simulink model "test"  (R2023b)
settings: Solver=FixedStepAuto  StartTime=0.0  StopTime=10.0  FixedStep=5e-8  RelTol=1e-3
undefined symbols (not defined in the file): powergui, sps_lib
libraries: spsMosfetLib x6, mcbcontrolslib x4, dspfdesign x3, slpidlib x3, simulink x2, spsDCVoltageSourceLib x1, spsPermanentMagnetSynchronousMachineLib x1, spsSawtoothGeneratorLib x1
settings Model: Creator=LZQ  LastModifiedBy=LZQ

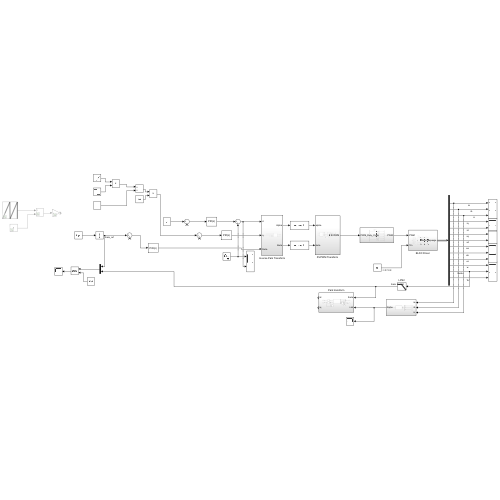
[thumbnail: Simulink's stored preview of the top-level diagram]
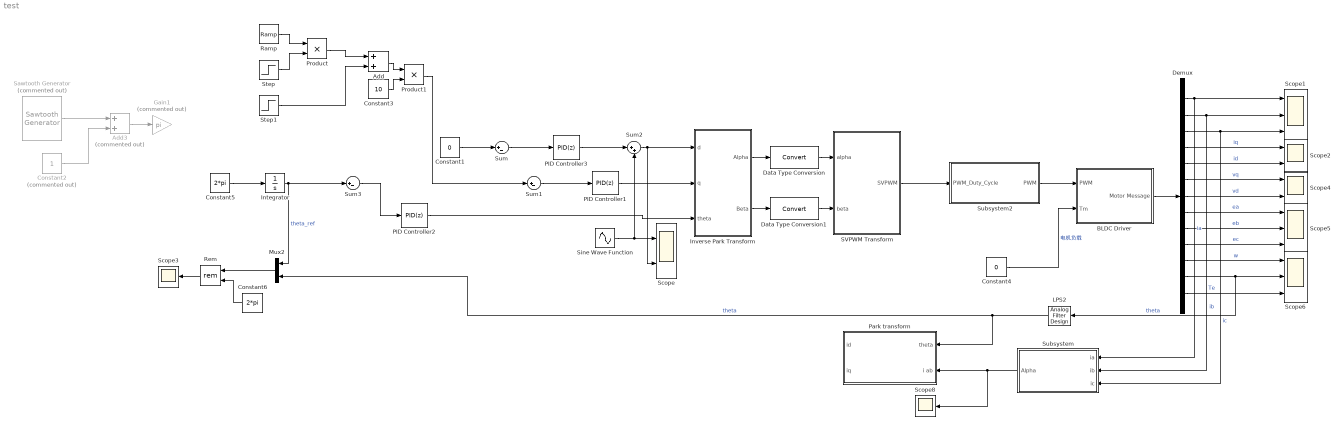
== system test ==
  Add : Sum
  Add3 : Sum  Commented=on
  BLDC Driver : Subsystem
  Constant1 : Constant  Value=0
  Constant2 : Constant  Commented=on
  Constant3 : Constant  Value=10
  Constant4 : Constant  Value=0
  Constant5 : Constant  Value=2*pi
  Constant6 : Constant  Value=2*pi
  Data Type Conversion : DataTypeConversion  SaturateOnIntegerOverflow=off  RndMeth=Floor
  Data Type Conversion1 : DataTypeConversion  SaturateOnIntegerOverflow=off  RndMeth=Floor
  Demux : Demux  Outputs=13
  Gain1 : Gain  Commented=on  Gain=pi
  Integrator : Integrator
  Inverse Park Transform : Subsystem
  LPS2 : dspfdesign/Analog Filter Design  method=Butterworth  filttype=Lowpass  N=8  Wlo=30  Whi=80  Rp=2  Rs=40
  Mux2 : Mux  Inputs=2
  PID Controller1 : slpidlib/PID Controller  Controller=PID  Form=Parallel  TimeDomain=Discrete-time  UseExternalTs=off  SampleTime=0.0005  IntegratorMethod=Forward Euler  FilterMethod=Forward Euler  ControllerParametersSource=internal  P=0.04  I=0.01  UseKiTs=off  D=0.008  N=100  UseFilter=on  TunerSelectOption=Transfer Function Based (PID Tuner App)  InitialConditionSource=internal  InitialConditionForIntegrator=0  InitialConditionForFilter=0  DifferentiatorICPrevScaledInput=0  ExternalReset=none  TrackingMode=off  Kt=1  LimitOutput=off  SatLimitsSource=internal  UpperSaturationLimit=inf  LowerSaturationLimit=-inf  LinearizeAsGain=on  AntiWindupMode=none  Kb=1  LimitIntegrator=off  UpperIntegratorSaturationLimit=inf  LowerIntegratorSaturationLimit=-inf  POutMin=[]  POutMax=[]  IOutMin=[-5]  IOutMax=[5]  DOutMin=[]  DOutMax=[]  NOutMin=[]  NOutMax=[]  SumOutMin=[-10]  SumOutMax=[10]  SaturationOutMin=[]  SaturationOutMax=[]  PParamMin=[]  PParamMax=[]  IParamMin=[]  IParamMax=[]  DParamMin=[]  DParamMax=[]  NParamMin=[]  NParamMax=[]  KbParamMin=[]  KbParamMax=[]  KtParamMin=[]  KtParamMax=[]  KbOutMin=[]  KbOutMax=[]  KtOutMin=[]  KtOutMax=[]  IntegratorOutMin=[]  IntegratorOutMax=[]  FilterOutMin=[]  FilterOutMax=[]  SumI1OutMin=[]  SumI1OutMax=[]  SumI2OutMin=[]  SumI2OutMax=[]  SumI3OutMin=[]  SumI3OutMax=[]  SumI4OutMin=[]  SumI4OutMax=[]  SumDOutMin=[]  SumDOutMax=[]  DifferentiatorOutMin=[]  DifferentiatorOutMax=[]  FilterDiffOutCoefMin=[]  FilterDiffOutCoefMax=[]  ReciprocalOutMin=[]  ReciprocalOutMax=[]  SumDenOutMin=[]  SumDenOutMax=[]  SumNumOutMin=[]  SumNumOutMax=[]  DivideOutMin=[]  DivideOutMax=[]  UdiffTsProdOutMin=[]  UdiffTsProdOutMax=[]  NTsProdOutMin=[]  NTsProdOutMax=[]  UintegralTsProdOutMin=[]  UintegralTsProdOutMax=[]  UngainTsProdOutMin=[]  UngainTsProdOutMax=[]  ClampingZeroOutDataTypeStr=Inherit: Inherit via back propagation  ClampingZeroOutMin=[]  ClampingZeroOutMax=[]  FilterDenConstantOutDataTypeStr=Inherit: Inherit via back propagation  FilterDenConstantOutMin=[]  FilterDenConstantOutMax=[]  PCopyOutDataTypeStr=Inherit: Inherit via back propagation  PCopyOutMin=[]  PCopyOutMax=[]  NCopyOutDataTypeStr=Inherit: Inherit via back propagation  NCopyOutMin=[]  NCopyOutMax=[]  IntegratorContinuousStateAttributes=''  IntegratorStateMustResolveToSignalObject=off  IntegratorRTWStateStorageClass=Auto  FilterContinuousStateAttributes=''  FilterStateMustResolveToSignalObject=off  FilterRTWStateStorageClass=Auto  ParallelPVariant=InternalParameters  IdealPVariant=Disabled  IVariant=InternalParameters  DVariant=InternalParameters  IntegratorVariant=Discrete  SatVariant=Disabled  AWVariant=Passthrough  PCopyVariant=Disabled  TRVariant=Disabled  FdbkBlocksVariant=Forward  IdealPFdbkVariant=Disabled  SatFdbkVariant=Disabled  DerivativeFilterVariant=ForwardEulerFilter  NVariant=InternalParameters  NCopyVariant=Disabled  FilterICVariant=InternalICsFilter  IntegratorICVariant=InternalICs  ExternalResetVariant=Disabled  TRSumVariant=Passthrough  SumFdbkVariant=Disabled  SumVariant=Sum_PID  TsampFilterVariant=InternalTs  TsampNgainVariant=Passthrough  TsampIntegralVariant=Disabled_SignalSpec  ExternalSaturationOutDataTypeStr=Inherit: Same as second input
  PID Controller2 : slpidlib/PID Controller  Controller=PID  Form=Parallel  TimeDomain=Discrete-time  UseExternalTs=off  SampleTime=0.0005  IntegratorMethod=Forward Euler  FilterMethod=Forward Euler  ControllerParametersSource=internal  P=0.1  I=0.04  UseKiTs=off  D=0  N=100  UseFilter=on  TunerSelectOption=Transfer Function Based (PID Tuner App)  InitialConditionSource=internal  InitialConditionForIntegrator=0  InitialConditionForFilter=0  DifferentiatorICPrevScaledInput=0  ExternalReset=none  TrackingMode=off  Kt=1  LimitOutput=off  SatLimitsSource=internal  UpperSaturationLimit=inf  LowerSaturationLimit=-inf  LinearizeAsGain=on  AntiWindupMode=none  Kb=1  LimitIntegrator=off  UpperIntegratorSaturationLimit=inf  LowerIntegratorSaturationLimit=-inf  POutMin=[]  POutMax=[]  IOutMin=[]  IOutMax=[]  DOutMin=[]  DOutMax=[]  NOutMin=[]  NOutMax=[]  SumOutMin=[]  SumOutMax=[]  SaturationOutMin=[]  SaturationOutMax=[]  PParamMin=[]  PParamMax=[]  IParamMin=[]  IParamMax=[]  DParamMin=[]  DParamMax=[]  NParamMin=[]  NParamMax=[]  KbParamMin=[]  KbParamMax=[]  KtParamMin=[]  KtParamMax=[]  KbOutMin=[]  KbOutMax=[]  KtOutMin=[]  KtOutMax=[]  IntegratorOutMin=[]  IntegratorOutMax=[]  FilterOutMin=[]  FilterOutMax=[]  SumI1OutMin=[]  SumI1OutMax=[]  SumI2OutMin=[]  SumI2OutMax=[]  SumI3OutMin=[]  SumI3OutMax=[]  SumI4OutMin=[]  SumI4OutMax=[]  SumDOutMin=[]  SumDOutMax=[]  DifferentiatorOutMin=[]  DifferentiatorOutMax=[]  FilterDiffOutCoefMin=[]  FilterDiffOutCoefMax=[]  ReciprocalOutMin=[]  ReciprocalOutMax=[]  SumDenOutMin=[]  SumDenOutMax=[]  SumNumOutMin=[]  SumNumOutMax=[]  DivideOutMin=[]  DivideOutMax=[]  UdiffTsProdOutMin=[]  UdiffTsProdOutMax=[]  NTsProdOutMin=[]  NTsProdOutMax=[]  UintegralTsProdOutMin=[]  UintegralTsProdOutMax=[]  UngainTsProdOutMin=[]  UngainTsProdOutMax=[]  ClampingZeroOutDataTypeStr=Inherit: Inherit via back propagation  ClampingZeroOutMin=[]  ClampingZeroOutMax=[]  FilterDenConstantOutDataTypeStr=Inherit: Inherit via back propagation  FilterDenConstantOutMin=[]  FilterDenConstantOutMax=[]  PCopyOutDataTypeStr=Inherit: Inherit via back propagation  PCopyOutMin=[]  PCopyOutMax=[]  NCopyOutDataTypeStr=Inherit: Inherit via back propagation  NCopyOutMin=[]  NCopyOutMax=[]  IntegratorContinuousStateAttributes=''  IntegratorStateMustResolveToSignalObject=off  IntegratorRTWStateStorageClass=Auto  FilterContinuousStateAttributes=''  FilterStateMustResolveToSignalObject=off  FilterRTWStateStorageClass=Auto  ParallelPVariant=InternalParameters  IdealPVariant=Disabled  IVariant=InternalParameters  DVariant=InternalParameters  IntegratorVariant=Discrete  SatVariant=Disabled  AWVariant=Passthrough  PCopyVariant=Disabled  TRVariant=Disabled  FdbkBlocksVariant=Forward  IdealPFdbkVariant=Disabled  SatFdbkVariant=Disabled  DerivativeFilterVariant=ForwardEulerFilter  NVariant=InternalParameters  NCopyVariant=Disabled  FilterICVariant=InternalICsFilter  IntegratorICVariant=InternalICs  ExternalResetVariant=Disabled  TRSumVariant=Passthrough  SumFdbkVariant=Disabled  SumVariant=Sum_PID  TsampFilterVariant=InternalTs  TsampNgainVariant=Passthrough  TsampIntegralVariant=Disabled_SignalSpec  ExternalSaturationOutDataTypeStr=Inherit: Same as second input
  PID Controller3 : slpidlib/PID Controller  Controller=PID  Form=Parallel  TimeDomain=Discrete-time  UseExternalTs=off  SampleTime=0.0005  IntegratorMethod=Forward Euler  FilterMethod=Forward Euler  ControllerParametersSource=internal  P=0.04  I=0.01  UseKiTs=off  D=0.008  N=100  UseFilter=on  TunerSelectOption=Transfer Function Based (PID Tuner App)  InitialConditionSource=internal  InitialConditionForIntegrator=0  InitialConditionForFilter=0  DifferentiatorICPrevScaledInput=0  ExternalReset=none  TrackingMode=off  Kt=1  LimitOutput=off  SatLimitsSource=internal  UpperSaturationLimit=inf  LowerSaturationLimit=-inf  LinearizeAsGain=on  AntiWindupMode=none  Kb=1  LimitIntegrator=off  UpperIntegratorSaturationLimit=inf  LowerIntegratorSaturationLimit=-inf  POutMin=[]  POutMax=[]  IOutMin=[-5]  IOutMax=[5]  DOutMin=[]  DOutMax=[]  NOutMin=[]  NOutMax=[]  SumOutMin=[-10]  SumOutMax=[10]  SaturationOutMin=[]  SaturationOutMax=[]  PParamMin=[]  PParamMax=[]  IParamMin=[]  IParamMax=[]  DParamMin=[]  DParamMax=[]  NParamMin=[]  NParamMax=[]  KbParamMin=[]  KbParamMax=[]  KtParamMin=[]  KtParamMax=[]  KbOutMin=[]  KbOutMax=[]  KtOutMin=[]  KtOutMax=[]  IntegratorOutMin=[]  IntegratorOutMax=[]  FilterOutMin=[]  FilterOutMax=[]  SumI1OutMin=[]  SumI1OutMax=[]  SumI2OutMin=[]  SumI2OutMax=[]  SumI3OutMin=[]  SumI3OutMax=[]  SumI4OutMin=[]  SumI4OutMax=[]  SumDOutMin=[]  SumDOutMax=[]  DifferentiatorOutMin=[]  DifferentiatorOutMax=[]  FilterDiffOutCoefMin=[]  FilterDiffOutCoefMax=[]  ReciprocalOutMin=[]  ReciprocalOutMax=[]  SumDenOutMin=[]  SumDenOutMax=[]  SumNumOutMin=[]  SumNumOutMax=[]  DivideOutMin=[]  DivideOutMax=[]  UdiffTsProdOutMin=[]  UdiffTsProdOutMax=[]  NTsProdOutMin=[]  NTsProdOutMax=[]  UintegralTsProdOutMin=[]  UintegralTsProdOutMax=[]  UngainTsProdOutMin=[]  UngainTsProdOutMax=[]  ClampingZeroOutDataTypeStr=Inherit: Inherit via back propagation  ClampingZeroOutMin=[]  ClampingZeroOutMax=[]  FilterDenConstantOutDataTypeStr=Inherit: Inherit via back propagation  FilterDenConstantOutMin=[]  FilterDenConstantOutMax=[]  PCopyOutDataTypeStr=Inherit: Inherit via back propagation  PCopyOutMin=[]  PCopyOutMax=[]  NCopyOutDataTypeStr=Inherit: Inherit via back propagation  NCopyOutMin=[]  NCopyOutMax=[]  IntegratorContinuousStateAttributes=''  IntegratorStateMustResolveToSignalObject=off  IntegratorRTWStateStorageClass=Auto  FilterContinuousStateAttributes=''  FilterStateMustResolveToSignalObject=off  FilterRTWStateStorageClass=Auto  ParallelPVariant=InternalParameters  IdealPVariant=Disabled  IVariant=InternalParameters  DVariant=InternalParameters  IntegratorVariant=Discrete  SatVariant=Disabled  AWVariant=Passthrough  PCopyVariant=Disabled  TRVariant=Disabled  FdbkBlocksVariant=Forward  IdealPFdbkVariant=Disabled  SatFdbkVariant=Disabled  DerivativeFilterVariant=ForwardEulerFilter  NVariant=InternalParameters  NCopyVariant=Disabled  FilterICVariant=InternalICsFilter  IntegratorICVariant=InternalICs  ExternalResetVariant=Disabled  TRSumVariant=Passthrough  SumFdbkVariant=Disabled  SumVariant=Sum_PID  TsampFilterVariant=InternalTs  TsampNgainVariant=Passthrough  TsampIntegralVariant=Disabled_SignalSpec  ExternalSaturationOutDataTypeStr=Inherit: Same as second input
  Park transform : Subsystem
  Product : Product
  Product1 : Product
  Ramp : simulink/Sources/Ramp  slope=0.2  start=0  InitialOutput=0.2
  Rem : Math  Operator=rem
  SVPWM Transform : Subsystem
  Sawtooth Generator : spsSawtoothGeneratorLib/Sawtooth Generator  Commented=on  Freq=1  Phase=360  Ts=0
  Scope : Scope  NumInputPorts=2
  Scope1 : Scope  NumInputPorts=3
  Scope2 : Scope  NumInputPorts=2
  Scope3 : Scope
  Scope4 : Scope  NumInputPorts=2
  Scope5 : Scope  NumInputPorts=3
  Scope6 : Scope  NumInputPorts=3
  Scope8 : Scope
  Sine Wave Function : Sin  Frequency=2*pi*2000  Phase=pi/2  SampleTime=0.000005
  Step : Step  Time=4  Before=1  After=0  SampleTime=0
  Step1 : Step  Time=4  SampleTime=0
  Subsystem : Subsystem
  Subsystem2 : Subsystem
  Sum : Sum  Inputs=|+-
  Sum1 : Sum  Inputs=|+-
  Sum2 : Sum  Inputs=|++
  Sum3 : Sum  Inputs=|+-
  wires:
  Product/1 -> Add/1
  PID Controller2/1 -> Inverse Park Transform/3(theta)
  Constant5/1 -> Integrator/1
  Demux/12 -> LPS2/1, Scope6/2  "theta"
  Demux/8 -> Scope5/1  "ea"
  Demux/5 -> Scope2/2  "id"
  Data Type Conversion/1 -> SVPWM Transform/1(alpha)
  Demux/3 -> Subsystem/3(ic), Scope1/3  "ic"
  Demux/9 -> Scope5/2  "eb"
  SVPWM Transform/1(SVPWM) -> Subsystem2/1(PWM_Duty_Cycle)
  Constant1/1 -> Sum/1
  Integrator/1 -> Mux2/1, Sum3/1  "theta_ref"
  Constant4/1 -> BLDC Driver/2(Tm)  "电机负载"
  Sum3/1 -> PID Controller2/1
  PID Controller3/1 -> Sum2/1
  Constant3/1 -> Product1/2
  Sum1/1 -> PID Controller1/1
  Subsystem/1(Alpha) -> Park transform/2(i ab), Scope8/1
  BLDC Driver/1(Motor Message) -> Demux/1
  Constant2/1 -> Add3/2
  Demux/11 -> Scope6/1  "w"
  Sum/1 -> PID Controller3/1
  Demux/1 -> Subsystem/1(ia), Scope1/1  "ia"
  Data Type Conversion1/1 -> SVPWM Transform/2(beta)
  Demux/7 -> Scope4/2  "vd"
  Add3/1 -> Gain1/1
  Demux/4 -> Scope2/1  "iq"
  Product1/1 -> Sum1/1
  Demux/10 -> Scope5/3  "ec"
  Step/1 -> Product/2
  Sum2/1 -> Inverse Park Transform/1(d), Scope/2
  Demux/13 -> Scope6/3  "Te"
  Subsystem2/1(PWM) -> BLDC Driver/1(PWM)
  LPS2/1 -> Mux2/2, Park transform/1(theta)  "theta"
  Rem/1 -> Scope3/1
  PID Controller1/1 -> Inverse Park Transform/2(q)
  Step1/1 -> Add/2
  Constant6/1 -> Rem/2
  Ramp/1 -> Product/1
  Inverse Park Transform/2(Beta) -> Data Type Conversion1/1
  Demux/2 -> Subsystem/2(ib), Scope1/2  "ib"
  Mux2/1 -> Rem/1
  Add/1 -> Product1/1
  Inverse Park Transform/1(Alpha) -> Data Type Conversion/1
  Sawtooth Generator/1 -> Add3/1
  Sine Wave Function/1 -> Sum2/2, Scope/1
  Demux/6 -> Scope4/1  "vq"

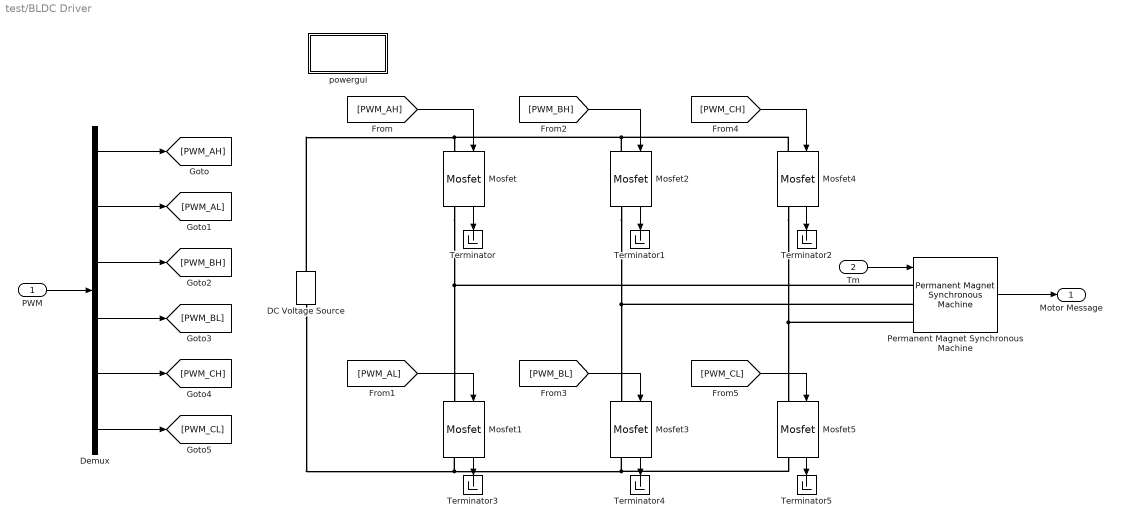
== system test/BLDC Driver ==
  PWM : Inport
  Tm : Inport  Port=2
  DC Voltage Source : spsDCVoltageSourceLib/DC Voltage Source  Amplitude=100  Measurements=Voltage
  Demux : Demux  Outputs=6
  Mosfet{,1..5} (6 alike) : spsMosfetLib/Mosfet  Ron=0.1  Lon=0  Rd=0.01  Vfd=0  IC=0  Rs=1e5  Cs=inf  Measurements=on
  Permanent Magnet Synchronous Machine : spsPermanentMagnetSynchronousMachineLib/Permanent Magnet Synchronous Machine  NbPhases=3  FluxDistribution=Sinusoidal  RotorType=Round  MechanicalLoad=Torque Tm  PresetModel=No  ShowDetailedParameters=on  MeasurementBus=off  Resistance=0.0485  Inductance=8.5e-3  dqInductances=[8.5e-3,8.5e-3]  La=0.000395  MachineConstant=Flux linkage established by magnets (V.s)  Flux=0.1194  VoltageCst=86.6271  TorqueCst=0.7164  Flat=120  Mechanical=[0.0027 0.0004924 4 0]  PolePairs=4  InitialConditions=[0,0, 0,0]  InitialConditions5ph=[0 0 0 0 0 0]  RefAngle=90 degrees behind phase A axis (modified Park)  IterativeDiscreteModel=Trapezoidal non iterative  TsBlock=-1  TsPowergui=0
  Terminator{,1..5} (6 alike) : Terminator
  powergui : Subsystem  Priority=1  AncestorBlock=sps_lib/powergui  DialogController=POWERSYS.PowerSysDialog  InitFcn=powergui( 'InitFcn_Callback' , gcb , 0 , [ ] );  mask(PSB option menu block){SimulationMode=Discrete, SampleTime=5e-8, frequency=60, Iterations=50, frequencyindice=0, Pbase=100e6, ErrMax=1e-4, UnitsV=kV, UnitsW=MW, buscounter=0, FunctionMessages=off, echomessages=off, EnableUseOfTLC=off, CurrentSourceSwitches=off, DisableSnubberDevices=off, DisableRonSwitches=off, DisableVfSwitches=off, DisplayEquations=off, AutomaticDiscreteSolvers=off, SolverType=Tustin/Backward Euler (TBE), Interpol=off, ExternalGateDelay=off, methode=off, Ts=100, x0status=blocks, SPID=on, SwTol=0, HookPort=off, NonlinearTolerance=1e-4, nMaxIteration=100, ContinueOnMaxIteration=off, RestoreLinks=warning, ResistiveCurrentMeasurement=off, Frange=[0:2:500], Ylog=off, Xlog=on, ShowGrid=off, save=off, variable=ZData, structure=0, ZoomFFT=off, StartTime=0.0, cycles=1, DisplayStyle=1, fundamental=60, FreqAxis=off, MaxFrequency=1000, frequencyindicesteady=1, RmsSteady=1, display=off}
      mask prompts: SimulationMode "Simulation type:"; SampleTime "Sample time (s):"; frequency "Frequency (Hz):"; Iterations "Max iterations"; frequencyindice "Frequency (Hz)"; Pbase "Base power (VA)"; ErrMax "PQ tolerance (pu)"; UnitsV "Voltage units"; UnitsW "Power units"; buscounter "Load flow bus counter"; FunctionMessages "Disable Specialized Power Systems warnings"; echomessages "Display Specialized Power Systems compilation messages"; EnableUseOfTLC "Use TLC file when in Accelerator Simulation Mode and for code generation"; CurrentSourceSwitches "Disable ideal switching"; DisableSnubberDevices "Disable snubbers in switching devices"; DisableRonSwitches "Disable Ron resistances in switching devices"; DisableVfSwitches "Disable forward voltages in switching devices"; DisplayEquations "Display circuit differential equations"; AutomaticDiscreteSolvers "Automatically handle Discrete solver and Advanced tab solver settings of blocks"; SolverType "Discrete solver"; Interpol "Interpolate switching events"; ExternalGateDelay "Use time-stamped gate signals"; methode "Store switching topologies"; Ts "Buffer size (MBytes):"; x0status "Start simulation with initial electrical states from:"; SPID "Use ideal switching devices"; SwTol "Switch tolerance"; HookPort "Allow multiple powergui blocks"; NonlinearTolerance "Solver tolerance"; nMaxIteration "Maximum number of iterations"; ContinueOnMaxIteration "Continue Simulation if maximum number of iterations is reached"; RestoreLinks "Restore disabled links of Simscape Power Systems ST blocks:"; ResistiveCurrentMeasurement "Use non ideal current measurement blocks (1e-4Ohm internal resistance)"; Frange "Frequency Range"; Ylog "Log impedance"; Xlog "log Frequency"; ShowGrid "grid"; save "Save Data To Workspace"; variable "Variable Name"; structure "Structure Name (PSBFFTSCOPE)"; ZoomFFT "ZoomFFT (PSBFFTSCOPE)"; StartTime "Start Time (PSBFFTSCOPE)"; cycles "Cycles (PSBFFTSCOPE)"; DisplayStyle "Display style (PSBFFTSCOPE)"; fundamental "Fundamental (PSBFFTSCOPE)"; FreqAxis "Frequency Axis (PSBFFTSCOPE)"; MaxFrequency "Max Frequency (PSBFFTSCOPE)"; frequencyindicesteady "Frequency indice (STEADYSTATE)"; RmsSteady "RMS display (STEADYSTATE)"; display "Display Results"
      mask help: Set simulation type, simulation parameters, and preferences.
      mask init:
      | dispMessage = '';
      | dispMessage = powergui('MaskInitialization',gcb,SimulationMode,SampleTime);
      settings: LibrarySourceBlock=sps_lib/powergui  PreSaveFcn=powergui( 'PreSaveFcn_Callback' , gcb , [ ] , [ ] );  OpenFcn=sps_rtmsupport('OpenFcn',gcbh)
      mask Help: helpview(psbhelp)
      mask TypeOptions SimulationMode: Continuous | Discrete | Phasor | Discrete phasor
      mask Callback SimulationMode: powergui('SimulationType',[],[],gcb);
      mask TypeOptions UnitsV: V | kV
      mask TypeOptions UnitsW: W | kW | MW
      mask Callback CurrentSourceSwitches: powergui('SimulationType',[],[],gcb);
      mask Callback AutomaticDiscreteSolvers: powergui('SimulationType',[],[],gcb);
      mask TypeOptions SolverType: Tustin/Backward Euler (TBE) | Tustin | Backward Euler
      mask Callback SolverType: powergui('SimulationType',[],[],gcb);
      mask Callback Interpol: powergui('SimulationType',[],[],gcb);
      mask Callback ExternalGateDelay: powergui('SimulationType',[],[],gcb);
      mask Callback methode: powergui('SimulationType',[],[],gcb);
      mask TypeOptions x0status: blocks | steady | zero
      mask TypeOptions RestoreLinks: yes | warning | no
      mask Callback display: sps_rtmsupport('parametereditingmodes',gcbh) % Will be executed last in parameter callbacks to ensure mask enable consistency
      mask DialogControl SolverTab Prompt: Solver
      mask DialogControl AutoSolverNote Prompt: The Simulation type parameter is governed by Simulink. To access the Powergui solver settings, unselect auto (Automatic solver selection) solver in the Simulink solver options.
      mask DialogControl Apps Prompt: Apps
      mask DialogControl StateAnalyzer Prompt: Measurements and States Analyzer
      mask DialogControl StateAnalyzer Callback: powerStates(bdroot(gcb))
      mask DialogControl LineParameterCalculator Prompt: Line Parameter Calculator
      mask DialogControl LineParameterCalculator Callback:
      | close_system(gcb)
      | powerLineParameters
      mask DialogControl CableParameterCalculator Prompt: Cable Parameter Calculator
      mask DialogControl CableParameterCalculator Callback:
      | close_system(gcb)
      | powerCableParameters
      mask DialogControl LineDecoupler Prompt: Line Decoupler
      mask DialogControl LineDecoupler Tooltip: Click to replace selected Distributed Parameters Line blocks with Decoupling Line blocks
      mask DialogControl LineDecoupler Callback:
      | close_system(gcb);
      | DecouplingLineReplace(gcs)
      mask DialogControl LoadFlowAnalyzer Prompt: Load Flow Analyzer
      mask DialogControl LoadFlowAnalyzer Callback:
      | close_system(gcb)
      | powerLoadFlow
      mask DialogControl LoadFlowParameters Prompt: Load Flow Parameters
      mask DialogControl ImpedanceCalculator Prompt: Impedance Calculator
      mask DialogControl ImpedanceCalculator Callback:
      | close_system(gcb);
      | powerImpedance(bdroot(gcs));
      mask DialogControl FFTAnalyzer Prompt: FFT Analyzer
      mask DialogControl FFTAnalyzer Callback:
      | close_system(gcb)
      | power_fftscope(bdroot(gcb),gcb)
      mask DialogControl LinearSystemAnalyzer Prompt: Linear System Analyzer
      mask DialogControl LinearSystemAnalyzer Callback:
      | close_system(gcb)
      | power_ltiview(bdroot(gcb))
      mask DialogControl HysteresisDesigner Prompt: Hysteresis Designer
      mask DialogControl HysteresisDesigner Callback:
      | close_system(gcb)
      | powerHysteresis('hysteresis.mat')
      mask DialogControl BlockCustomizer Prompt: Block Customizer
      mask DialogControl BlockCustomizer Callback:
      | close_system(gcb);
      | power_customize;
      mask DialogControl ReportGenerator Prompt: Report Generator
      mask DialogControl ReportGenerator Callback:
      | close_system(gcb)
      | power_report(bdroot(gcb))
      mask DialogControl obsolete Prompt: ...
      mask DialogControl MachineInitialization Prompt: Machine Initialization
      mask DialogControl MachineInitialization Callback:
      | close_system(gcb)
      | powericon('machineInitTool',bdroot(gcb),gcb)
      mask DialogControl Preferences Prompt: Preferences
      mask DialogControl Solver Prompt: Solver
      mask DialogControl SolverDetails Prompt: Solver details for nonlinear elements
      mask Display: color('blue'),disp(dispMessage)
  Motor Message : Outport
  wires:
  [PWM_AH] -> Mosfet/1
  Mosfet/1 -> Terminator/1
  Mosfet2/1 -> Terminator1/1
  Mosfet4/1 -> Terminator2/1
  Mosfet1/1 -> Terminator3/1
  Mosfet3/1 -> Terminator4/1
  Mosfet5/1 -> Terminator5/1
  [PWM_BH] -> Mosfet2/1
  [PWM_BL] -> Mosfet3/1
  [PWM_AL] -> Mosfet1/1
  [PWM_CH] -> Mosfet4/1
  [PWM_CL] -> Mosfet5/1
  PWM/1 -> Demux/1
  Demux/1 -> [PWM_AH]
  Demux/2 -> [PWM_AL]
  Demux/3 -> [PWM_BH]
  Demux/4 -> [PWM_BL]
  Demux/5 -> [PWM_CH]
  Demux/6 -> [PWM_CL]
  Permanent Magnet Synchronous Machine/1 -> Motor Message/1
  Tm/1 -> Permanent Magnet Synchronous Machine/1
  connections:
  Mosfet2/RConn1 -- Permanent Magnet Synchronous Machine/LConn2 -- Mosfet3/LConn1
  Mosfet/RConn1 -- Permanent Magnet Synchronous Machine/LConn1 -- Mosfet1/LConn1
  Mosfet4/RConn1 -- Mosfet5/LConn1 -- Permanent Magnet Synchronous Machine/LConn3
  DC Voltage Source/RConn1 -- Mosfet4/LConn1 -- Mosfet2/LConn1 -- Mosfet/LConn1
  DC Voltage Source/LConn1 -- Mosfet5/RConn1 -- Mosfet3/RConn1 -- Mosfet1/RConn1

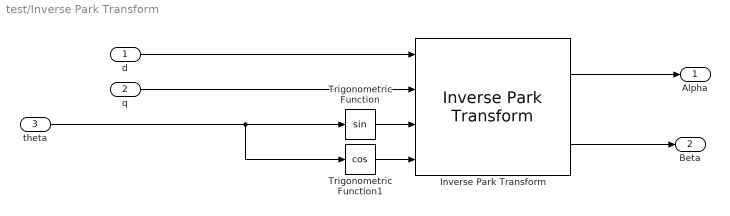
== system test/Inverse Park Transform ==
  d : Inport
  q : Inport  Port=2
  theta : Inport  Port=3
  Inverse Park Transform : mcbcontrolslib/Inverse Park Transform  PhaseInput=Two inputs  AxisAlignment=D-axis  ThetaInput=Sine and Cosine electrical position  AngleInput=Per-unit  N_points=1024
      settings: LibrarySourceBlock=mcblib/Controls/Math Transforms/Inverse Park Transform
  Trigonometric Function : Trigonometry
  Trigonometric Function1 : Trigonometry  Operator=cos
  Alpha : Outport
  Beta : Outport  Port=2
  wires:
  theta/1 -> Trigonometric Function1/1, Trigonometric Function/1
  Trigonometric Function1/1 -> Inverse Park Transform/4
  Trigonometric Function/1 -> Inverse Park Transform/3
  Inverse Park Transform/1 -> Alpha/1
  d/1 -> Inverse Park Transform/1
  q/1 -> Inverse Park Transform/2
  Inverse Park Transform/2 -> Beta/1

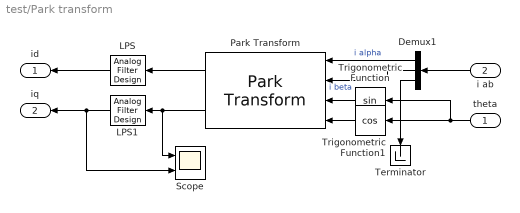
== system test/Park transform ==
  theta : Inport
  i ab : Inport  Port=2
  Demux1 : Demux  Outputs=3
  LPS : dspfdesign/Analog Filter Design  method=Butterworth  filttype=Lowpass  N=3  Wlo=500  Whi=80  Rp=2  Rs=40
  LPS1 : dspfdesign/Analog Filter Design  method=Butterworth  filttype=Lowpass  N=3  Wlo=500  Whi=80  Rp=2  Rs=40
  Park Transform : mcbcontrolslib/Park Transform  PhaseInput=Two inputs  AxisAlignment=D-axis  ThetaInput=Sine and Cosine electrical position  AngleInput=Per-unit  N_points=1024
      settings: LibrarySourceBlock=mcblib/Controls/Math Transforms/Park Transform
  Scope : Scope  NumInputPorts=2
  Terminator : Terminator
  Trigonometric Function : Trigonometry
  Trigonometric Function1 : Trigonometry  Operator=cos
  id : Outport
  iq : Outport  Port=2
  wires:
  Demux1/3 -> Terminator/1
  Trigonometric Function1/1 -> Park Transform/4
  theta/1 -> Trigonometric Function/1, Trigonometric Function1/1
  Park Transform/1 -> LPS/1
  LPS/1 -> id/1
  Park Transform/2 -> Scope/1, LPS1/1
  Demux1/2 -> Park Transform/2  "i beta"
  Demux1/1 -> Park Transform/1  "i alpha"
  Trigonometric Function/1 -> Park Transform/3
  i ab/1 -> Demux1/1
  LPS1/1 -> iq/1, Scope/2

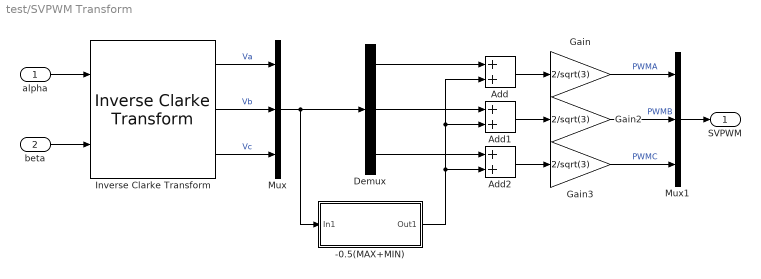
== system test/SVPWM Transform ==
  alpha : Inport
  beta : Inport  Port=2
  -0.5(MAX+MIN) : Subsystem
  Add : Sum
  Add1 : Sum
  Add2 : Sum
  Demux : Demux  Outputs=3
  Gain : Gain  Gain=2/sqrt(3)
  Gain2 : Gain  Gain=2/sqrt(3)
  Gain3 : Gain  Gain=2/sqrt(3)
  Inverse Clarke Transform : mcbcontrolslib/Inverse Clarke Transform  PhaseInput=Two inputs  EnPowerInv=off
      settings: LibrarySourceBlock=mcblib/Controls/Math Transforms/Inverse Clarke Transform
  Mux : Mux  Inputs=3
  Mux1 : Mux  Inputs=3
  SVPWM : Outport
  wires:
  -0.5(MAX+MIN)/1(Out1) -> Add2/2, Add1/2, Add/2
  Mux/1 -> -0.5(MAX+MIN)/1(In1), Demux/1
  Inverse Clarke Transform/1 -> Mux/1  "Va"
  Demux/2 -> Add1/1
  Add/1 -> Gain/1
  Inverse Clarke Transform/2 -> Mux/2  "Vb"
  Add2/1 -> Gain3/1
  Inverse Clarke Transform/3 -> Mux/3  "Vc"
  Demux/1 -> Add/1
  Demux/3 -> Add2/1
  Add1/1 -> Gain2/1
  alpha/1 -> Inverse Clarke Transform/1
  beta/1 -> Inverse Clarke Transform/2
  Gain2/1 -> Mux1/2  "PWMB"
  Gain/1 -> Mux1/1  "PWMA"
  Gain3/1 -> Mux1/3  "PWMC"
  Mux1/1 -> SVPWM/1

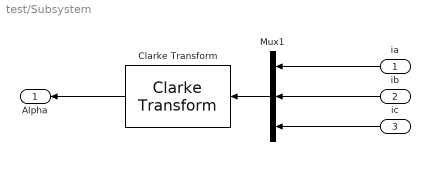
== system test/Subsystem ==
  ia : Inport
  ib : Inport  Port=2
  ic : Inport  Port=3
  Clarke Transform : mcbcontrolslib/Clarke Transform  VariantControl=Variant2  PhaseInput=Three inputs  EnPowerInv=off
      settings: LibrarySourceBlock=mcblib/Controls/Math Transforms/Clarke Transform
  Mux1 : Mux  Inputs=3
  Alpha : Outport
  wires:
  Mux1/1 -> Clarke Transform/1
  ia/1 -> Mux1/1
  ib/1 -> Mux1/2
  Clarke Transform/1 -> Alpha/1
  ic/1 -> Mux1/3

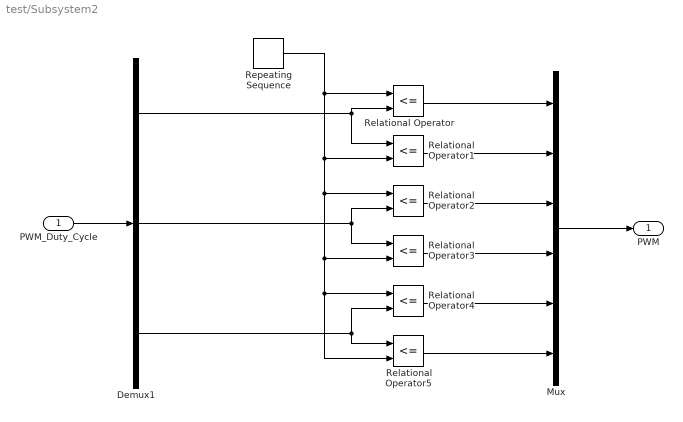
== system test/Subsystem2 ==
  PWM_Duty_Cycle : Inport  OutDataTypeStr=double  PortDimensions=3  SampleTime=[4.9999999999999998e-08,0]
  Demux1 : Demux  Outputs=3
  Mux : Mux  Inputs=6
  Relational Operator{,1..5} (6 alike) : RelationalOperator  Operator=<=  OutDataTypeStr=boolean  RndMeth=Simplest  InputSameDT=off
  Repeating Sequence : simulink/Sources/Repeating Sequence  rep_seq_t=[0 0.00005]  rep_seq_y=[-50 50]
  PWM : Outport  OutDataTypeStr=boolean  PortDimensions=6  SampleTime=0
  wires:
  Relational Operator3/1 -> Mux/4
  Relational Operator4/1 -> Mux/5
  Demux1/3 -> Relational Operator5/1, Relational Operator4/2
  Relational Operator2/1 -> Mux/3
  Demux1/2 -> Relational Operator3/1, Relational Operator2/2
  Demux1/1 -> Relational Operator1/1, Relational Operator/2
  PWM_Duty_Cycle/1 -> Demux1/1
  Repeating Sequence/1 -> Relational Operator/1, Relational Operator1/2, Relational Operator2/1, Relational Operator3/2, Relational Operator4/1, Relational Operator5/2
  Mux/1 -> PWM/1
  Relational Operator5/1 -> Mux/6
  Relational Operator/1 -> Mux/1
  Relational Operator1/1 -> Mux/2

== system test/BLDC Driver/powergui ==
  note: Graphical user interface for the analysis of
      | Simscape Power Systems (Specialized Technology) circuits.
      | Place the Powergui block in the top-level of your model and double-click
      | on it to open the GUI.
  EquivalentModel1 : Subsystem
      mask init:
      | S  = GetDataForEquivalentModel('Discrete',gcbh);
      mask Display:
      | color('red')
      | disp('EQUIVALENT CIRCUIT\nDiscrete')
  Ground : Ground
  Terminator : Terminator
  wires:
  Ground/1 -> Terminator/1

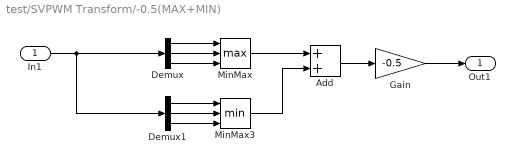
== system test/SVPWM Transform/-0.5(MAX+MIN) ==
  In1 : Inport
  Add : Sum
  Demux : Demux  Outputs=3
  Demux1 : Demux  Outputs=3
  Gain : Gain  Gain=-0.5
  MinMax : MinMax  Function=max  Inputs=3
  MinMax3 : MinMax  Inputs=3
  Out1 : Outport
  wires:
  In1/1 -> Demux1/1, Demux/1
  Demux/1 -> MinMax/1
  Demux/2 -> MinMax/2
  Demux/3 -> MinMax/3
  Demux1/1 -> MinMax3/1
  Demux1/2 -> MinMax3/2
  Demux1/3 -> MinMax3/3
  MinMax/1 -> Add/1
  MinMax3/1 -> Add/2
  Add/1 -> Gain/1
  Gain/1 -> Out1/1

== system test/BLDC Driver/powergui/EquivalentModel1 ==
  Gates : Subsystem
  Sources : Subsystem
  State-Space : S-Function  FunctionName=sfun_spssw_discc  Parameters=S.Ts,S.A, S.B, S.C, S.D, S.x0, S.EnableUseOfTLC,S.SwitchResistance ,S.SwitchType, S.SwitchGateInitialValue, S.OutputsToResetToZero, S.TBEON,S.SaveMatrices,S.BufferSize  SFunctionDeploymentMode=off  EnableBusSupport=off
  Status : Subsystem
  Yout : Subsystem
  wires:
  Gates/1(gates) -> State-Space/2
  Sources/1(u) -> State-Space/1
  State-Space/2 -> Status/1(status)
  State-Space/1 -> Yout/1(v,i)

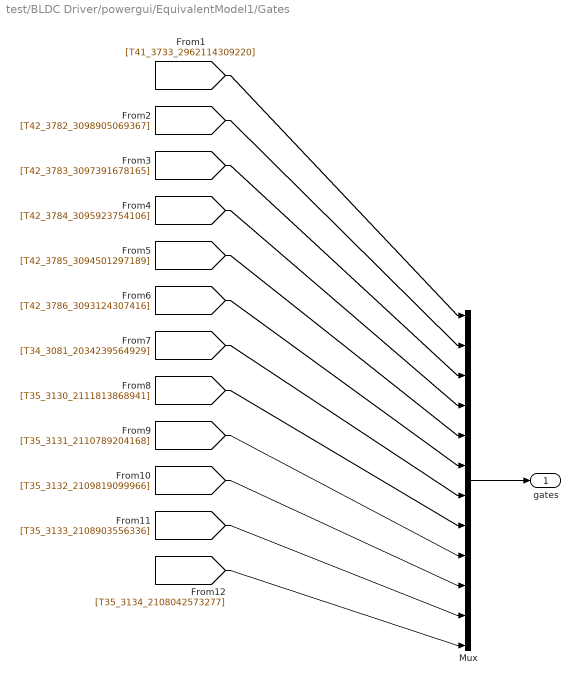
== system test/BLDC Driver/powergui/EquivalentModel1/Gates ==
  Mux : Mux  Inputs=[1 1 1 1 1 1 1 1 1 1 1 1]
  gates : Outport  VectorParamsAs1DForOutWhenUnconnected=off
  wires:
  Mux/1 -> gates/1
  [T41_3733_2962114309220] -> Mux/1
  [T42_3782_3098905069367] -> Mux/2
  [T42_3783_3097391678165] -> Mux/3
  [T42_3784_3095923754106] -> Mux/4
  [T42_3785_3094501297189] -> Mux/5
  [T42_3786_3093124307416] -> Mux/6
  [T34_3081_2034239564929] -> Mux/7
  [T35_3130_2111813868941] -> Mux/8
  [T35_3131_2110789204168] -> Mux/9
  [T35_3132_2109819099966] -> Mux/10
  [T35_3133_2108903556336] -> Mux/11
  [T35_3134_2108042573277] -> Mux/12

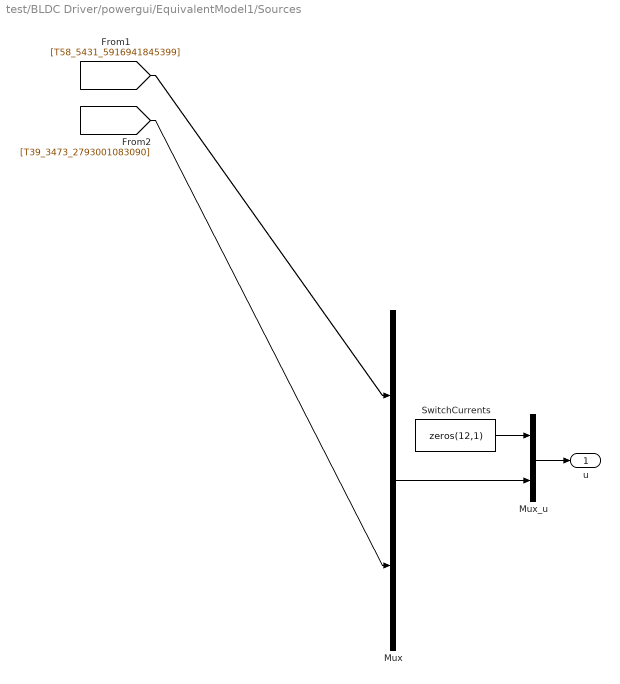
== system test/BLDC Driver/powergui/EquivalentModel1/Sources ==
  Mux : Mux  Inputs=[2 1]
  Mux_u : Mux  Inputs=[12 3]
  SwitchCurrents : Constant  Value=zeros(12,1)
  u : Outport  VectorParamsAs1DForOutWhenUnconnected=off
  wires:
  Mux_u/1 -> u/1
  SwitchCurrents/1 -> Mux_u/1
  Mux/1 -> Mux_u/2
  [T58_5431_5916941845399] -> Mux/1
  [T39_3473_2793001083090] -> Mux/2

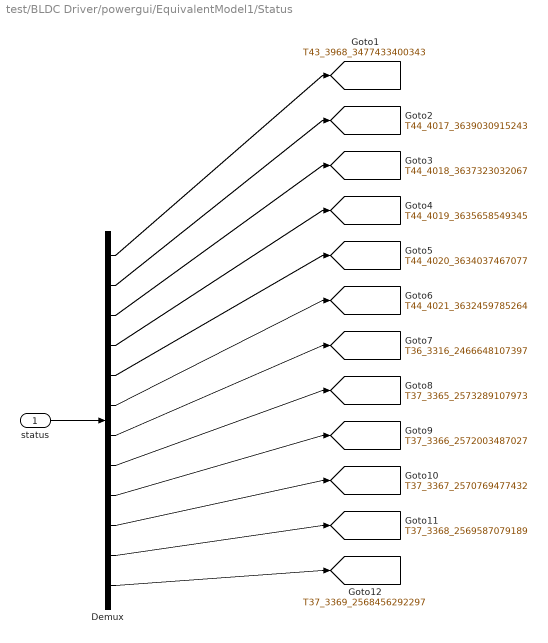
== system test/BLDC Driver/powergui/EquivalentModel1/Status ==
  status : Inport
  Demux : Demux  Outputs=[1 1 1 1 1 1 1 1 1 1 1 1]
  tag scope: T36_3316_2466648107397=global, T37_3365_2573289107973=global, T37_3366_2572003487027=global, T37_3367_2570769477432=global, T37_3368_2569587079189=global, T37_3369_2568456292297=global, T43_3968_3477433400343=global, T44_4017_3639030915243=global, T44_4018_3637323032067=global, T44_4019_3635658549345=global, T44_4020_3634037467077=global, T44_4021_3632459785264=global
  wires:
  status/1 -> Demux/1
  Demux/1 -> [T43_3968_3477433400343]
  Demux/2 -> [T44_4017_3639030915243]
  Demux/3 -> [T44_4018_3637323032067]
  Demux/4 -> [T44_4019_3635658549345]
  Demux/5 -> [T44_4020_3634037467077]
  Demux/6 -> [T44_4021_3632459785264]
  Demux/7 -> [T36_3316_2466648107397]
  Demux/8 -> [T37_3365_2573289107973]
  Demux/9 -> [T37_3366_2572003487027]
  Demux/10 -> [T37_3367_2570769477432]
  Demux/11 -> [T37_3368_2569587079189]
  Demux/12 -> [T37_3369_2568456292297]

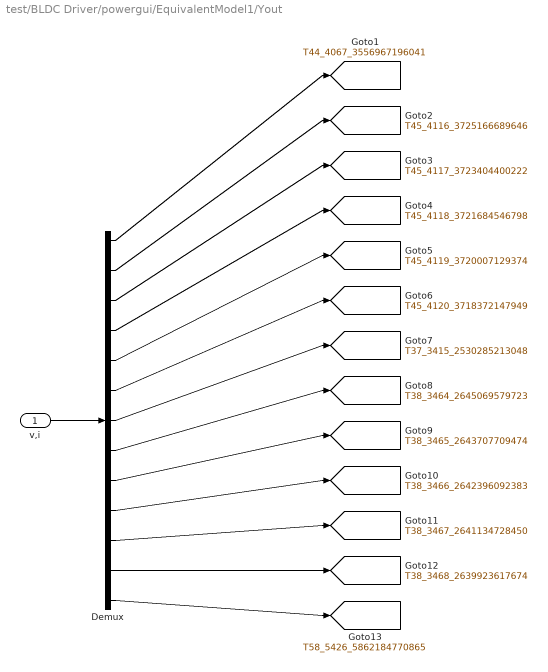
== system test/BLDC Driver/powergui/EquivalentModel1/Yout ==
  v,i : Inport
  Demux : Demux  Outputs=[1 1 1 1 1 1 1 1 1 1 1 1 2]
  tag scope: T37_3415_2530285213048=global, T38_3464_2645069579723=global, T38_3465_2643707709474=global, T38_3466_2642396092383=global, T38_3467_2641134728450=global, T38_3468_2639923617674=global, T44_4067_3556967196041=global, T45_4116_3725166689646=global, T45_4117_3723404400222=global, T45_4118_3721684546798=global, T45_4119_3720007129374=global, T45_4120_3718372147949=global, T58_5426_5862184770865=global
  wires:
  v,i/1 -> Demux/1
  Demux/1 -> [T44_4067_3556967196041]
  Demux/2 -> [T45_4116_3725166689646]
  Demux/3 -> [T45_4117_3723404400222]
  Demux/4 -> [T45_4118_3721684546798]
  Demux/5 -> [T45_4119_3720007129374]
  Demux/6 -> [T45_4120_3718372147949]
  Demux/7 -> [T37_3415_2530285213048]
  Demux/8 -> [T38_3464_2645069579723]
  Demux/9 -> [T38_3465_2643707709474]
  Demux/10 -> [T38_3466_2642396092383]
  Demux/11 -> [T38_3467_2641134728450]
  Demux/12 -> [T38_3468_2639923617674]
  Demux/13 -> [T58_5426_5862184770865]
